simulink model "sf_spectrum_analyzer"  (R2017b)
settings: Solver=ode5  StartTime=0.0  StopTime=Inf  FixedStep=1e-4  MaxStep=1e-4  RelTol=1e-3  EnableMultiTasking=on
settings Model: Creator=The MathWorks, Inc.  LastModifiedBy=The MathWorks, Inc.
settings DataIOCC: SaveFormat=Array
settings OptimizationCC: ExpressionDepthLimit=2147483647  InitFltsAndDblsToZero=on  EfficientMapNaN2IntZero=off  LifeSpan=1
settings DebuggingCC: UnderspecifiedInitializationDetection=Classic  MergeDetectMultiDrivingBlocksExec=none  SolverPrmCheckMsg=warning  FcnCallInpInsideContextMsg=warning  StateNameClashWarn=warning  SFUnexpectedBacktrackingDiag=warning  SFNoUnconditionalDefaultTransitionDiag=warning  SFExecutionAtInitializationDiag=none
settings HardwareCC: ProdBitPerPointer=32  ProdBitPerSizeT=32  ProdBitPerPtrDiffT=32  ProdLargestAtomicFloat=None  ProdIntDivRoundTo=Undefined  ProdEndianess=Unspecified  ProdWordSize=32  ProdHWDeviceType=32-bit Generic
settings ModelReferenceCC: PropagateSignalLabelsOutOfModel=off
settings SFSimCC: SimParseCustomCode=off  MATLABDynamicMemAlloc=off
settings RTWCC: SystemTargetFile=ert.tlc  TemplateMakefile=ert_default_tmf  Description=Real-Time Workshop Embedded Coder (no auto configuration)  GenerateReport=on  IncludeHyperlinkInReport=on  LaunchReport=on  GenerateTraceInfo=on  GenerateTraceReport=on  GenerateTraceReportSl=on  GenerateTraceReportSf=on  GenerateTraceReportEml=on
settings CodeAppCC: IgnoreCustomStorageClasses=off  CustomSymbolStrType=$N$R$M  StateflowObjectComments=on  InternalIdentifier=Classic
settings ERTTargetCC: MultiwordLength=2048  GenerateSampleERTMain=on  SupportContinuousTime=on  ERTCustomFileTemplate=example_file_process.tlc  ConvertIfToSwitch=off  SuppressUnreachableDefaultCases=off
settings ConfigComp: CovMetricSettings=dw  CovHtmlReporting=on  CovSaveCumulativeToWorkspaceVar=on  CovSaveSingleToWorkspaceVar=on  CovExternalEMLEnable=off  CovSFcnEnable=off

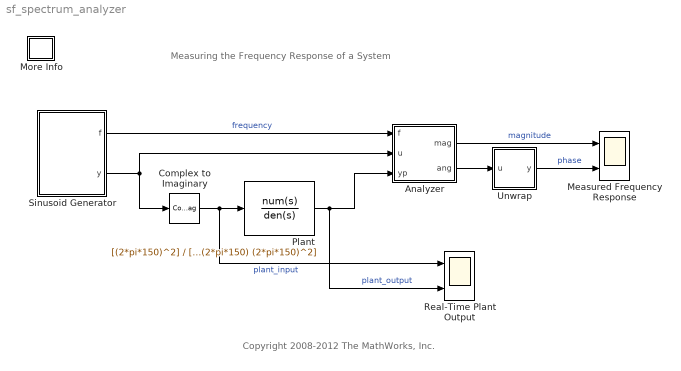
== system sf_spectrum_analyzer ==
  note: Copyright 2008-2012 The MathWorks, Inc.
  note: Measuring the Frequency Response of a System
  Analyzer : Stateflow chart  TreatAsAtomicUnit=on
  Complex to Imaginary : ComplexToRealImag  Output=Imag
  Measured Frequency Response : Scope  NumInputPorts=2
  More Info : Subsystem
      settings: OpenFcn=showdemo(bdroot(gcs))
      mask Display: disp('?')
  Plant : TransferFcn  Numerator=[(2*pi*150)^2]  Denominator=[1 2*0.3*(2*pi*150) (2*pi*150)^2]
  Real-Time Plant Output : Scope  NumInputPorts=2
  Sinusoid Generator : Subsystem  TreatAsAtomicUnit=on  mask{fstart=10, fstop=1000, fstep=10, delay=0.2}
      mask prompts: fstart "Initial frequency"; fstop "Stop frequency"; fstep "Step frequency"; delay "Delay at each frequency"
      mask help: Outputs a signal with constantly increasing frequency
  Unwrap : Stateflow chart  TreatAsAtomicUnit=on
  wires:
  Complex to Imaginary/1 -> Plant/1, Real-Time Plant Output/1  "plant_input"
  Plant/1 -> Analyzer/3(yp), Real-Time Plant Output/2  "plant_output"
  Analyzer/1(mag) -> Measured Frequency Response/1  "magnitude"
  Analyzer/2(ang) -> Unwrap/1(u)
  Sinusoid Generator/2(y) -> Complex to Imaginary/1, Analyzer/2(u)
  Sinusoid Generator/1(f) -> Analyzer/1(f)  "frequency"
  Unwrap/1(y) -> Measured Frequency Response/2  "phase"

== system sf_spectrum_analyzer/More Info ==

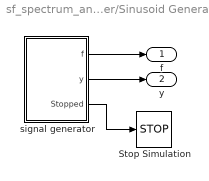
== system sf_spectrum_analyzer/Sinusoid Generator ==
  Stop Simulation : Stop
  signal generator : Stateflow chart  TreatAsAtomicUnit=on
  f : Outport
  y : Outport  Port=2
  wires:
  signal generator/2(y) -> y/1
  signal generator/1(f) -> f/1
  signal generator/3(" Stopped") -> Stop Simulation/1

== stateflow chart sf_spectrum_analyzer/Sinusoid Generator/signal generator ==
  state A
    en, du:
    t = temporalCount(sec);
    yprev = y;
    y = exp(2*pi*f*t*1j);
  state Stopped
  (default) -> A : {
      | f = fstart;
      | y = 0j;
      | }
  (junction 10) -> A [order 2]
  A -> (junction 10) : [after(delay,sec) && imag(yprev).*imag(y) <= 0 && imag(y) > 0]
      | {
      | f = f + fstep;
      | }
  (junction 10) -> Stopped [order 1] : [f > fstop]
  data: delay parameter double; f output; y output; yprev local; fstep parameter double; fstart parameter double; fstop parameter double; Stopped output boolean; t local

== stateflow chart sf_spectrum_analyzer/Analyzer ==
  state A
    en:
    y = 0j; yn = 0j;
    du:
    y = y + u.*yp;
    yn = yn + u.*imag(u);
  A -> A : [hasChanged(f)]
      | {
      | mag = abs(y)/abs(yn);
      | ang = -angle(y) + pi/2;
      | }
  data: f input; mag output; ang output; u input; y local; yn local; yp input

== stateflow chart sf_spectrum_analyzer/Unwrap ==
  state A
    en, du:
    y = u + offset;
    yprev = y;
  (default) -> A : {offset = 0;}
  A -> A [order 1] : [u+offset-yprev > pi]
      | { offset = offset - 2*pi; }
  A -> A [order 2] : [u+offset-yprev < -pi]
      | { offset = offset + 2*pi;}
  data: u input; y output; offset local; yprev local
